simulink subsystem "Power_Window_ECU"  (R2021a)
settings: Solver=VariableStepAuto  StartTime=0.0  StopTime=10.0  RelTol=1e-3
settings Model: Creator=achu  LastModifiedBy=Sai229

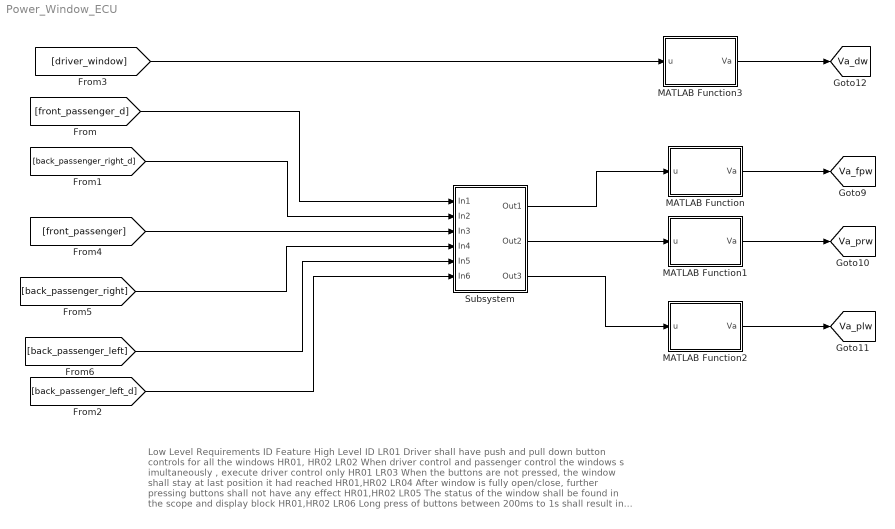
== system Power_Window_ECU ==
  note: Low Level Requirements
      |
      | ID
      | Feature
      | High Level ID
      |
      | LR01
      | Driver shall have push and pull down button controls for all the windows
      | HR01, HR02
      |
      | LR02
      | When driver control and passenger control the windows s imultaneously , execute driver control only
      | HR01
      |
      | LR03
      | When the buttons are not pressed, the window shall stay at last position it had reached
      | HR01,HR02
      |
      | LR04
      | After window is fully open/close, further pressing buttons shall not have any effect
      | HR01,HR02
      |
      | LR05
      | The status of the window shall be found in the scope and display block
      | HR01,HR02
      |
      | LR06
      | Long press of buttons between 200ms to 1s shall result in automatic pushing up or pulling down of window to max
      | HR01,HR02
      |
      | LR07
      | When lock is ON, only the driver shall have controls and passengers shall not be able to control the windows
      | HR03
  MATLAB Function : MATLAB Function  TreatAsAtomicUnit=on
  MATLAB Function1 : MATLAB Function  TreatAsAtomicUnit=on
  MATLAB Function2 : MATLAB Function  TreatAsAtomicUnit=on
  MATLAB Function3 : MATLAB Function  TreatAsAtomicUnit=on
  Subsystem : Subsystem
  tag scope: Va_dw=global, Va_fpw=global, Va_plw=global, Va_prw=global
  wires:
  MATLAB Function3/1(Va) -> [Va_dw]
  [driver_window] -> MATLAB Function3/1(u)
  MATLAB Function1/1(Va) -> [Va_prw]
  MATLAB Function/1(Va) -> [Va_fpw]
  MATLAB Function2/1(Va) -> [Va_plw]
  [front_passenger_d] -> Subsystem/1(In1)
  [back_passenger_right_d] -> Subsystem/2(In2)
  [front_passenger] -> Subsystem/3(In3)
  [back_passenger_right] -> Subsystem/4(In4)
  [back_passenger_left] -> Subsystem/5(In5)
  [back_passenger_left_d] -> Subsystem/6(In6)
  Subsystem/1(Out1) -> MATLAB Function/1(u)
  Subsystem/2(Out2) -> MATLAB Function1/1(u)
  Subsystem/3(Out3) -> MATLAB Function2/1(u)

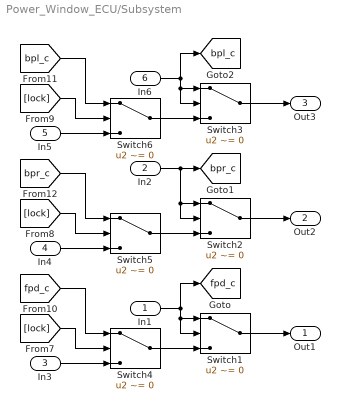
== system Power_Window_ECU/Subsystem ==
  In1 : Inport
  In2 : Inport  Port=2
  In3 : Inport  Port=3
  In4 : Inport  Port=4
  In5 : Inport  Port=5
  In6 : Inport  Port=6
  Switch{1..6} (6 alike) : Switch  Criteria=u2 ~= 0
  Out1 : Outport
  Out2 : Outport  Port=2
  Out3 : Outport  Port=3
  tag scope: bpl_c=global, bpr_c=global, fpd_c=global
  wires:
  Switch4/1 -> Switch1/3
  Switch1/1 -> Out1/1
  In6/1 -> [bpl_c], Switch3/1, Switch3/2
  [bpr_c] -> Switch5/1
  In5/1 -> Switch6/3
  [lock] -> Switch6/2
  Switch5/1 -> Switch2/3
  In1/1 -> [fpd_c], Switch1/1, Switch1/2
  [lock] -> Switch5/2
  [bpl_c] -> Switch6/1
  Switch6/1 -> Switch3/3
  [fpd_c] -> Switch4/1
  [lock] -> Switch4/2
  In4/1 -> Switch5/3
  Switch3/1 -> Out3/1
  In3/1 -> Switch4/3
  Switch2/1 -> Out2/1
  In2/1 -> [bpr_c], Switch2/1, Switch2/2

== matlab function Power_Window_ECU/MATLAB Function ==
  data: u input; Va output
function Va = fcn(u)
if (u==1)
    output=20;
elseif (u==-1)
    output=-20;
else
    output=0;
end
     
Va = output;

== matlab function Power_Window_ECU/MATLAB Function2 ==
  data: u input; Va output
function Va = fcn(u)
if (u==1)
    output=20;
elseif (u==-1)
    output=-20;
else
    output=0;
end
     
Va = output;

== matlab function Power_Window_ECU/MATLAB Function3 ==
  data: u input; Va output
function Va = fcn(u)
if (u==1)
    output=20;
elseif (u==-1)
    output=-20;
else
    output=0;
end
     
Va = output;

== matlab function Power_Window_ECU/MATLAB Function1 ==
  data: u input; Va output
function Va = fcn(u)
if (u==1)
    output=20;
elseif (u==-1)
    output=-20;
else
    output=0;
end
     
Va = output;
